simulink model "model2PID"  (R2022a)
settings: Solver=VariableStepAuto  StartTime=0.0  StopTime=10.0  RelTol=1e-3
libraries: simulink_extras x2
settings Model: Creator=Ekaterina  LastModifiedBy=Ekaterina

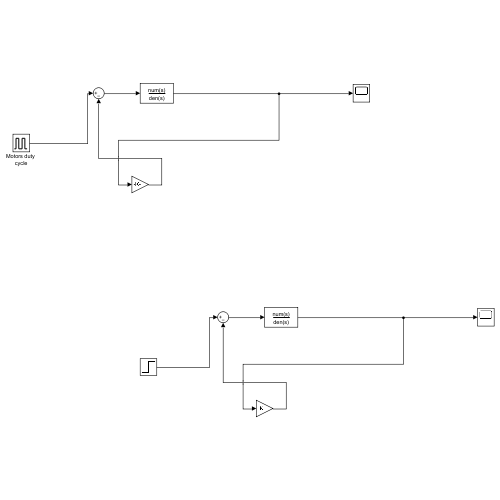
[thumbnail: Simulink's stored preview of the top-level diagram]
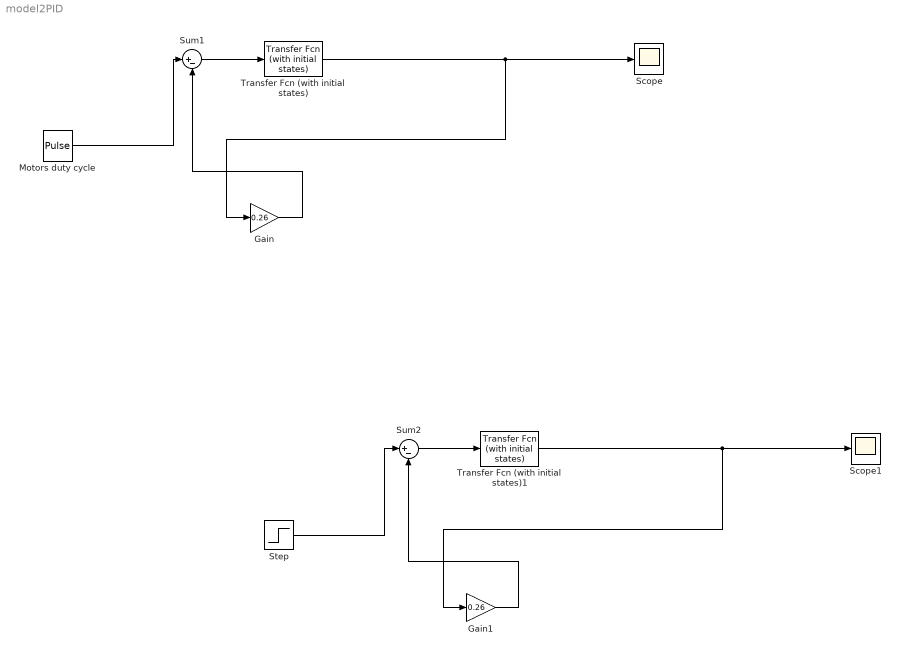
== system model2PID ==
  Gain : Gain  Gain=0.26
  Gain1 : Gain  Gain=0.26
  Motors duty cycle : DiscretePulseGenerator  PulseType=Time based  Period=10  PulseWidth=40
  Scope : Scope
  Scope1 : Scope
  Step : Step  SampleTime=100
  Sum1 : Sum  Inputs=|+-
  Sum2 : Sum  Inputs=|+-
  Transfer Fcn (with initial states) : simulink_extras/Additional Linear/Transfer Fcn (with initial states)  N=[0 0 8.914 5.959 ]  D="[1  0.4083 1.017 0.1075]"  X0=0
  Transfer Fcn (with initial states)1 : simulink_extras/Additional Linear/Transfer Fcn (with initial states)  N=[0 0 8.914 5.959 ]  D="[1  0.4083 1.017 0.1075]"  X0=0
  wires:
  Sum1/1 -> Transfer Fcn (with initial states)/1
  Transfer Fcn (with initial states)/1 -> Gain/1, Scope/1
  Gain/1 -> Sum1/2
  Motors duty cycle/1 -> Sum1/1
  Step/1 -> Sum2/1
  Gain1/1 -> Sum2/2
  Transfer Fcn (with initial states)1/1 -> Gain1/1, Scope1/1
  Sum2/1 -> Transfer Fcn (with initial states)1/1
